simulink model "logging_equivalent"  (R2021b)
settings: Solver=VariableStepAuto  StartTime=0.0  StopTime=10.0  RelTol=1e-3
libraries: simulink x4
settings Model: Creator=cemery  LastModifiedBy=cemery

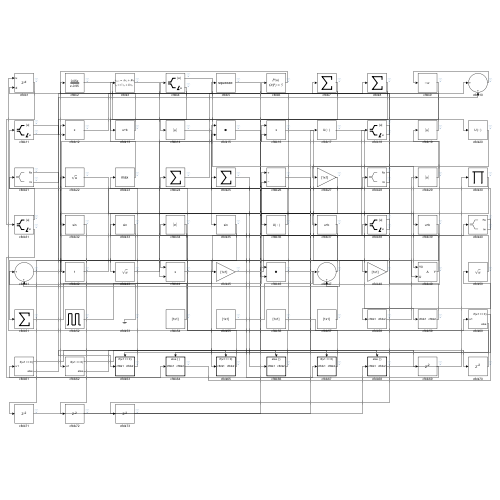
[thumbnail: Simulink's stored preview of the top-level diagram]
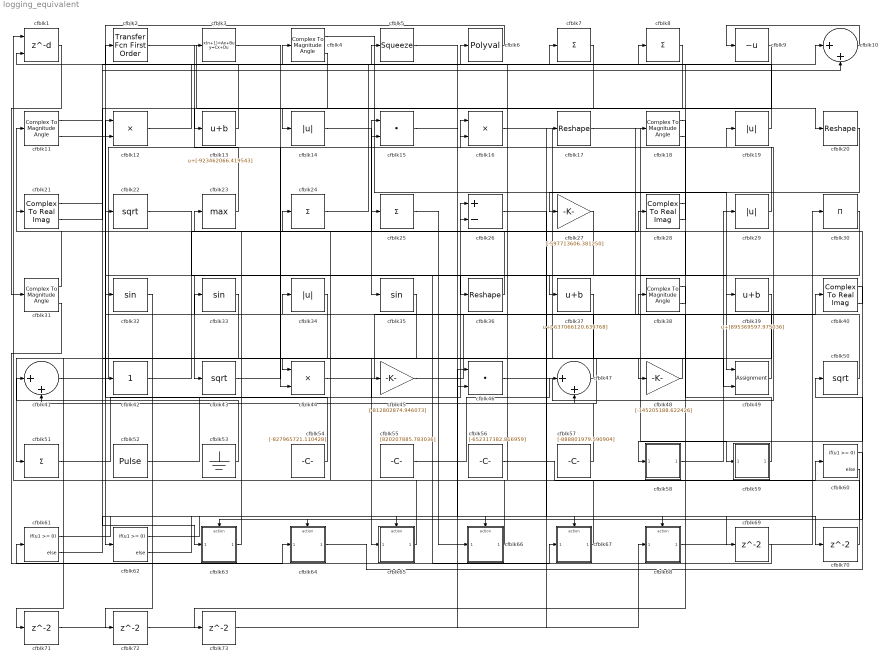
== system logging_equivalent ==
  cfblk1 : Delay  DelayLengthSource=Input port  SampleTime=1
      settings: InputPortMap=u0,p1
  cfblk10 : Sum  Inputs=|++
  cfblk{4,11,18,31,38} (5 alike) : ComplexToMagnitudeAngle
  cfblk12 : Product  Inputs=**
  cfblk13 : Bias  Bias=[-923462066.419543]
  cfblk{14,19,29,34} (4 alike) : Abs
  cfblk15 : DotProduct  InputSameDT=on  OutDataTypeStr=Inherit: Inherit via internal rule
  cfblk16 : Product  Inputs=**
  cfblk17 : Reshape
  cfblk2 : simulink/Discrete/Transfer Fcn First Order  PoleZ=0.95  ICPrevOutput=0.0  DoSatur=off
  cfblk20 : Reshape
  cfblk21 : ComplexToRealImag
  cfblk22 : Sqrt  SaturateOnIntegerOverflow=on
  cfblk23 : MinMax  Function=max
  cfblk{7..8,24..25,51} (5 alike) : Sum  Inputs=+
  cfblk26 : Sum  Inputs=+-
  cfblk27 : Gain  Gain=[-597713606.381250]
  cfblk28 : ComplexToRealImag
  cfblk3 : DiscreteStateSpace
  cfblk30 : Product  Inputs=*
  cfblk32 : Trigonometry
  cfblk33 : Trigonometry
  cfblk35 : Trigonometry
  cfblk36 : Reshape
  cfblk37 : Bias  Bias=[-637066120.639768]
  cfblk39 : Bias  Bias=[895369597.975036]
  cfblk40 : ComplexToRealImag
  cfblk41 : Sum  Inputs=|++
  cfblk42 : simulink/Math Operations/Slider Gain  gain=1  low=0  high=2
  cfblk43 : Sqrt  SaturateOnIntegerOverflow=on
  cfblk44 : Product  Inputs=**
  cfblk45 : Gain  Gain=[-812802874.946073]
  cfblk46 : DotProduct  InputSameDT=on  OutDataTypeStr=Inherit: Inherit via internal rule
  cfblk47 : Sum  Inputs=|++
  cfblk48 : Gain  Gain=[-145205188.622426]
  cfblk49 : Assignment  DiagnosticForDimensions=Warning  IndexOptions=Index vector (dialog)  Indices=1  OutputSizes=1
  cfblk5 : Squeeze
  cfblk50 : Sqrt  SaturateOnIntegerOverflow=on
  cfblk52 : DiscretePulseGenerator  PulseType=Time based  Amplitude=[-578887056.439533]  Period=[54917977.033567]  PulseWidth=5  PhaseDelay=[5.000000]
  cfblk53 : Ground
  cfblk54 : Constant  Value=[-827965721.110428]  SampleTime=1
  cfblk55 : Constant  Value=[820207885.783036]  SampleTime=1
  cfblk56 : Constant  Value=[-652317382.816959]  SampleTime=1
  cfblk57 : Constant  Value=[-888801979.590904]  SampleTime=1
  cfblk58 : Subsystem
  cfblk59 : Subsystem
  cfblk6 : Polyval  Coefs=[ +2.081618890e-019, -1.441693666e-014, +4.719686976e-010, -8.536869453e-006, +1.621573104e-001, -8.087801117e+001 ]
  cfblk60 : If  IfExpression=u1 >= 0  SampleTime=1
  cfblk61 : If  IfExpression=u1 >= 0  SampleTime=1
  cfblk62 : If  IfExpression=u1 >= 0  SampleTime=1
  cfblk63 : Subsystem  TreatAsAtomicUnit=on
  cfblk64 : Subsystem  TreatAsAtomicUnit=on
  cfblk65 : Subsystem  TreatAsAtomicUnit=on
  cfblk66 : Subsystem  TreatAsAtomicUnit=on
  cfblk67 : Subsystem  TreatAsAtomicUnit=on
  cfblk68 : Subsystem  TreatAsAtomicUnit=on
  cfblk{69..73} (5 alike) : Delay  SampleTime=1
  cfblk9 : UnaryMinus
  wires:
  cfblk35/1 -> cfblk65/1(cfblk1)
  cfblk25/1 -> cfblk66/1(cfblk1)
  cfblk4/1 -> cfblk49/1
  cfblk46/1 -> cfblk19/1
  cfblk14/1 -> cfblk67/1(cfblk1)
  cfblk6/1 -> cfblk62/1
  cfblk2/1 -> cfblk20/1
  cfblk17/1 -> cfblk59/1(cfblk1)
  cfblk31/1 -> cfblk11/1
  cfblk56/1 -> cfblk60/1
  cfblk27/1 -> cfblk43/1
  cfblk50/1 -> cfblk26/1
  cfblk36/1 -> cfblk15/1
  cfblk23/1 -> cfblk3/1
  cfblk54/1 -> cfblk12/1
  cfblk64/1(cfblk2) -> cfblk50/1
  cfblk67/1(cfblk2) -> cfblk16/1
  cfblk10/1 -> cfblk9/1
  cfblk42/1 -> cfblk28/1
  cfblk63/1(cfblk2) -> cfblk23/1
  cfblk45/1 -> cfblk40/1
  cfblk16/1 -> cfblk49/2
  cfblk8/1 -> cfblk12/2
  cfblk1/1 -> cfblk31/1
  cfblk4/2 -> cfblk14/1
  cfblk41/1 -> cfblk16/2
  cfblk37/1 -> cfblk51/1
  cfblk20/1 -> cfblk27/1
  cfblk34/1 -> cfblk42/1
  cfblk19/1 -> cfblk4/1
  cfblk3/1 -> cfblk35/1
  cfblk40/1 -> cfblk58/1(cfblk1)
  cfblk53/1 -> cfblk41/1
  cfblk68/1(cfblk2) -> cfblk30/1
  cfblk57/1 -> cfblk41/2
  cfblk48/1 -> cfblk44/1
  cfblk44/1 -> cfblk18/1
  cfblk47/1 -> cfblk33/1
  cfblk51/1 -> cfblk26/2
  cfblk22/1 -> cfblk39/1
  cfblk43/1 -> cfblk15/2
  cfblk65/1(cfblk2) -> cfblk24/1
  cfblk13/1 -> cfblk2/1
  cfblk15/1 -> cfblk37/1
  cfblk66/1(cfblk2) -> cfblk34/1
  cfblk49/1 -> cfblk22/1
  cfblk40/2 -> cfblk25/1
  cfblk29/1 -> cfblk6/1
  cfblk9/1 -> cfblk13/1
  cfblk18/1 -> cfblk32/1
  cfblk18/2 -> cfblk1/2
  cfblk21/1 -> cfblk48/1
  cfblk31/2 -> cfblk64/1(cfblk1)
  cfblk12/1 -> cfblk5/1
  cfblk52/1 -> cfblk45/1
  cfblk7/1 -> cfblk46/2
  cfblk58/1(cfblk2) -> cfblk29/1
  cfblk38/2 -> cfblk21/1
  cfblk30/1 -> cfblk44/2
  cfblk28/1 -> cfblk36/1
  cfblk21/2 -> cfblk10/1
  cfblk28/2 -> cfblk7/1
  cfblk55/1 -> cfblk47/1
  cfblk11/1 -> cfblk63/1(cfblk1)
  cfblk39/1 -> cfblk47/2
  cfblk59/1(cfblk2) -> cfblk38/1
  cfblk24/1 -> cfblk8/1
  cfblk11/2 -> cfblk10/2
  cfblk60/1 -> cfblk63/Action
  cfblk60/2 -> cfblk64/Action
  cfblk61/1 -> cfblk65/Action
  cfblk61/2 -> cfblk66/Action
  cfblk62/1 -> cfblk67/Action
  cfblk62/2 -> cfblk68/Action
  cfblk5/1 -> cfblk69/1
  cfblk69/1 -> cfblk61/1
  cfblk26/1 -> cfblk70/1
  cfblk70/1 -> cfblk1/1
  cfblk33/1 -> cfblk71/1
  cfblk71/1 -> cfblk46/1
  cfblk32/1 -> cfblk72/1
  cfblk72/1 -> cfblk68/1(cfblk1)
  cfblk38/1 -> cfblk73/1
  cfblk73/1 -> cfblk17/1

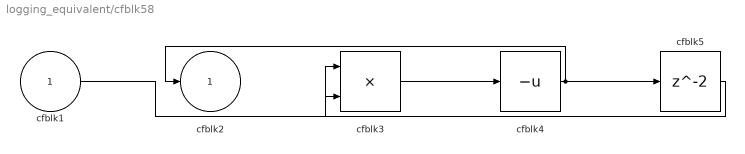
== system logging_equivalent/cfblk58 ==
  cfblk1 : Inport
  cfblk3 : Product
  cfblk4 : UnaryMinus
  cfblk5 : Delay  SampleTime=1
  cfblk2 : Outport
  wires:
  cfblk4/1 -> cfblk2/1, cfblk5/1
  cfblk1/1 -> cfblk3/1
  cfblk3/1 -> cfblk4/1
  cfblk5/1 -> cfblk3/2

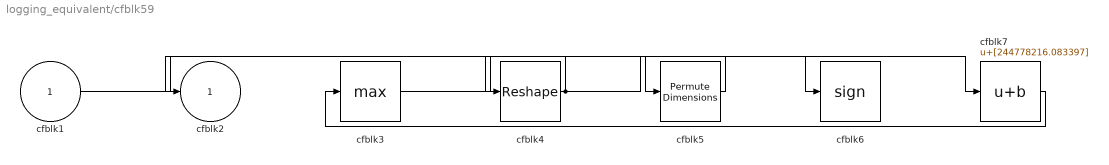
== system logging_equivalent/cfblk59 ==
  cfblk1 : Inport
  cfblk3 : MinMax  Function=max
  cfblk4 : Reshape
  cfblk5 : PermuteDimensions
  cfblk6 : Signum
  cfblk7 : Bias  Bias=[244778216.083397]
  cfblk2 : Outport
  wires:
  cfblk1/1 -> cfblk7/1
  cfblk7/1 -> cfblk3/1
  cfblk3/1 -> cfblk5/1
  cfblk4/1 -> cfblk2/1, cfblk6/1
  cfblk5/1 -> cfblk4/1

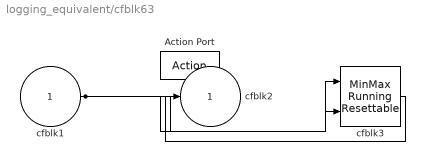
== system logging_equivalent/cfblk63 ==
  cfblk1 : Inport
  Action Port : ActionPort  ActionPortLabel=if(u1 >= 0)
  cfblk3 : simulink/Math Operations/MinMax Running Resettable  Function=min  vinit=0.0
  cfblk2 : Outport
  wires:
  cfblk1/1 -> cfblk3/1, cfblk3/2
  cfblk3/1 -> cfblk2/1

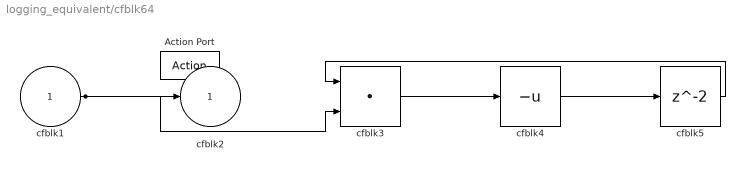
== system logging_equivalent/cfblk64 ==
  cfblk1 : Inport
  Action Port : ActionPort  ActionPortLabel=else
  cfblk3 : DotProduct  InputSameDT=on  OutDataTypeStr=Inherit: Inherit via internal rule
  cfblk4 : UnaryMinus
  cfblk5 : Delay
  cfblk2 : Outport
  wires:
  cfblk1/1 -> cfblk2/1, cfblk3/2
  cfblk3/1 -> cfblk4/1
  cfblk4/1 -> cfblk5/1
  cfblk5/1 -> cfblk3/1

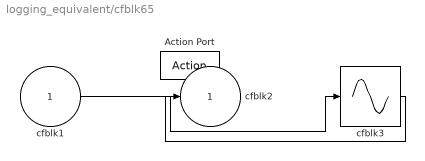
== system logging_equivalent/cfblk65 ==
  cfblk1 : Inport
  Action Port : ActionPort  ActionPortLabel=if(u1 >= 0)
  cfblk3 : Sin  TimeSource=Use external signal  SampleTime=0
  cfblk2 : Outport
  wires:
  cfblk1/1 -> cfblk3/1
  cfblk3/1 -> cfblk2/1

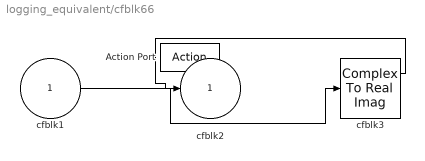
== system logging_equivalent/cfblk66 ==
  cfblk1 : Inport
  Action Port : ActionPort  ActionPortLabel=else
  cfblk3 : ComplexToRealImag
  cfblk2 : Outport
  wires:
  cfblk1/1 -> cfblk3/1
  cfblk3/1 -> cfblk2/1

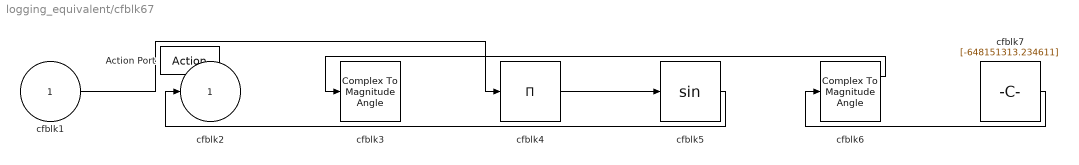
== system logging_equivalent/cfblk67 ==
  cfblk1 : Inport
  Action Port : ActionPort  ActionPortLabel=if(u1 >= 0)
  cfblk3 : ComplexToMagnitudeAngle
  cfblk4 : Product  Inputs=*
  cfblk5 : Trigonometry
  cfblk6 : ComplexToMagnitudeAngle
  cfblk7 : Constant  Value=[-648151313.234611]  SampleTime=1
  cfblk2 : Outport
  wires:
  cfblk5/1 -> cfblk2/1
  cfblk1/1 -> cfblk4/1
  cfblk4/1 -> cfblk5/1
  cfblk6/1 -> cfblk3/1
  cfblk7/1 -> cfblk6/1

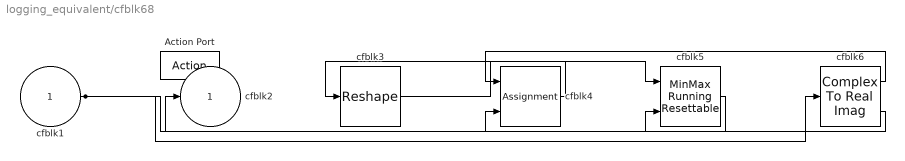
== system logging_equivalent/cfblk68 ==
  cfblk1 : Inport
  Action Port : ActionPort  ActionPortLabel=else
  cfblk3 : Reshape
  cfblk4 : Assignment  DiagnosticForDimensions=Warning  IndexOptions=Index vector (dialog)  Indices=1  OutputSizes=1
  cfblk5 : simulink/Math Operations/MinMax Running Resettable  Function=min  vinit=0.0
  cfblk6 : ComplexToRealImag
  cfblk2 : Outport
  wires:
  cfblk5/1 -> cfblk2/1
  cfblk1/1 -> cfblk6/1, cfblk4/2
  cfblk3/1 -> cfblk5/1
  cfblk6/1 -> cfblk4/1
  cfblk6/2 -> cfblk5/2
  cfblk4/1 -> cfblk3/1
